simulink model "AD_Terry_VV"  (R2020b)
settings: Solver=VariableStepAuto  StartTime=0.0  StopTime=10.0  RelTol=1e-3
values from neighbouring files (symbols this model uses):
  A_2 = zeros(3)    [ANGULARTUNEVERSION2_VandV.m]
  B_2 = I_inv    [ANGULARTUNEVERSION2_VandV.m]
  C_2 = eye(3)    [ANGULARTUNEVERSION2_VandV.m]
  C_D = 0.6    [ANGULARTUNEVERSION2_VandV.m]    (also in Drag_Model_VV.m)
  constant_v = 1    [ANGULARTUNEVERSION2_VandV.m]
  D_2 = zeros(3)    [ANGULARTUNEVERSION2_VandV.m]
  rho = 1.225    [ANGULARTUNEVERSION2_VandV.m]    (also in Drag_Model_VV.m)
  S = 1*1.8    (= 1.8)    [ANGULARTUNEVERSION2_VandV.m]    (also in Drag_Model_VV.m = 2.5)
  sine_v = 0    [ANGULARTUNEVERSION2_VandV.m]
  T = 10.5    [ANGULARTUNEVERSION2_VandV.m]
  theta_wanted = [pi/2; 0; 0]    [ANGULARTUNEVERSION2_VandV.m]
  v_vehicle = [20; 10; 0]    [ANGULARTUNEVERSION2_VandV.m]    (also in Drag_Model_VV.m = [2;3;4])
  x_amp = 10    [ANGULARTUNEVERSION2_VandV.m]
  x_cp = [0.3; 0.2; 0.4]    [ANGULARTUNEVERSION2_VandV.m]
  x_freq = 1    [ANGULARTUNEVERSION2_VandV.m]
  y_amp = 15    [ANGULARTUNEVERSION2_VandV.m]
  y_freq = 1    [ANGULARTUNEVERSION2_VandV.m]
  z_amp = 5    [ANGULARTUNEVERSION2_VandV.m]
  z_freq = 1    [ANGULARTUNEVERSION2_VandV.m]
libraries: mpclib x1, fuzblock x1, cstblocks x1
settings Model: Creator=Jonathan van Zyl  LastModifiedBy=Jonathan van Zyl

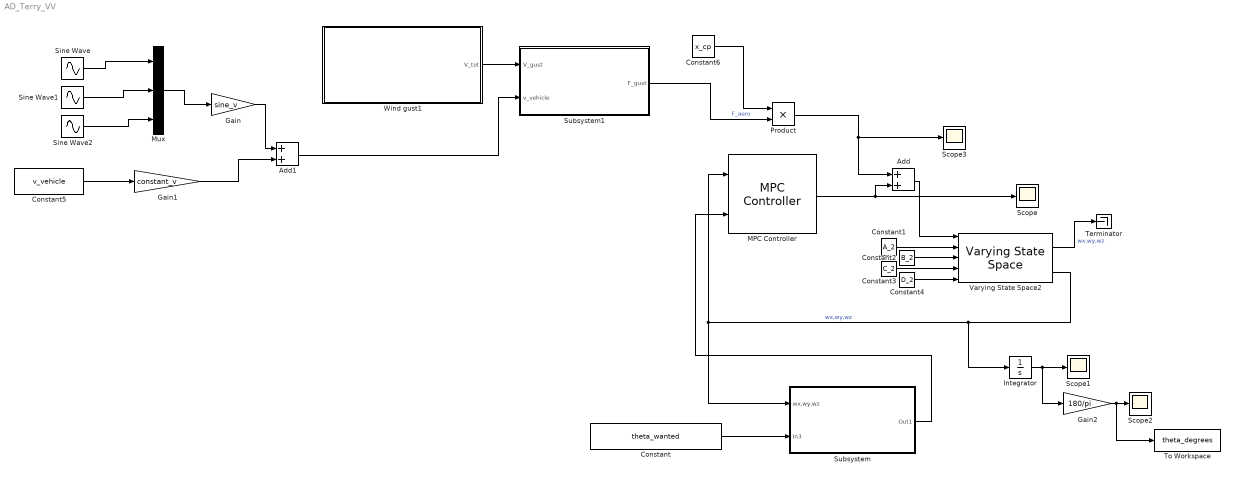
== system AD_Terry_VV ==
  Add : Sum
  Add1 : Sum
  Constant : Constant  Value=theta_wanted
  Constant1 : Constant  Value=A_2
  Constant2 : Constant  Value=B_2
  Constant3 : Constant  Value=C_2
  Constant4 : Constant  Value=D_2
  Constant5 : Constant  Value=v_vehicle
  Constant6 : Constant  Value=x_cp
  Gain : Gain  Gain=sine_v
  Gain1 : Gain  Gain=constant_v
  Gain2 : Gain  Gain=180/pi
  Integrator : Integrator
  MPC Controller : mpclib/MPC Controller  SCDEnableBlockLinearizationSpecification=on  mpcobj=MPCDesignerSession.AppData.Controllers.MPC  is_multiple=0  enable_value=0  return_u0=off  updateMPCinCallerWorkspace=on  md_inport=off  mv_inport=off  uref_inport=off  return_cost=off  return_mvseq=off  return_qpstatus=off  return_xseq=off  return_state=off  return_ovseq=off  state_inport=off  umin_inport=off  umax_inport=off  ymin_inport=off  ymax_inport=off  cc_inport=off  ywt_inport=off  uwt_inport=off  duwt_inport=off  rhoeps_inport=off  pm_inport=off  MaximumP=10  HorizonChoice=FixedHorizon  n_ts=0.1  n_p=10  n_mv=3  n_md=0  n_ud=0  n_mo=3  n_uo=0  BlockDataType=double  SampleTimeInherited=off  switch_inport=off
  Mux : Mux  Inputs=3
  Product : Product
  Scope{,1..3} (4 alike) : Scope
  Sine Wave : Sin  Amplitude=x_amp  Frequency=x_freq  SampleTime=0
  Sine Wave1 : Sin  Amplitude=y_amp  Frequency=y_freq  SampleTime=0
  Sine Wave2 : Sin  Amplitude=z_amp  Frequency=z_freq  SampleTime=0
  Subsystem : Subsystem
  Subsystem1 : Subsystem
  Terminator : Terminator
  To Workspace : ToWorkspace  VariableName=theta_degrees  SaveFormat=Timeseries  SampleTime=-1
  Varying State Space2 : cstblocks/Linear Parameter Varying/Varying State Space  x0=0  xNames=''  OutputX=on  OutputDX=off
  Wind gust1 : Subsystem
  wires:
  Constant5/1 -> Gain1/1
  Gain1/1 -> Add1/2
  Sine Wave/1 -> Mux/1
  Sine Wave1/1 -> Mux/2
  Sine Wave2/1 -> Mux/3
  Mux/1 -> Gain/1
  Gain/1 -> Add1/1
  Constant6/1 -> Product/1
  Subsystem1/1(F_gust) -> Product/2  "F_aero"
  Wind gust1/1(V_tot) -> Subsystem1/1(V_gust)
  Constant/1 -> Subsystem/2(In3)
  Varying State Space2/2 -> Integrator/1, MPC Controller/1, Subsystem/1(wx,wy,wz)  "wx,wy,wz"
  Constant1/1 -> Varying State Space2/2
  Subsystem/1(Out1) -> MPC Controller/2
  Integrator/1 -> Gain2/1, Scope1/1
  Constant3/1 -> Varying State Space2/4
  Constant2/1 -> Varying State Space2/3
  Product/1 -> Scope3/1, Add/1
  Gain2/1 -> To Workspace/1, Scope2/1
  Varying State Space2/1 -> Terminator/1  "wx,wy,wz"
  Add1/1 -> Subsystem1/2(v_vehicle)
  MPC Controller/1 -> Scope/1, Add/2
  Add/1 -> Varying State Space2/1
  Constant4/1 -> Varying State Space2/5

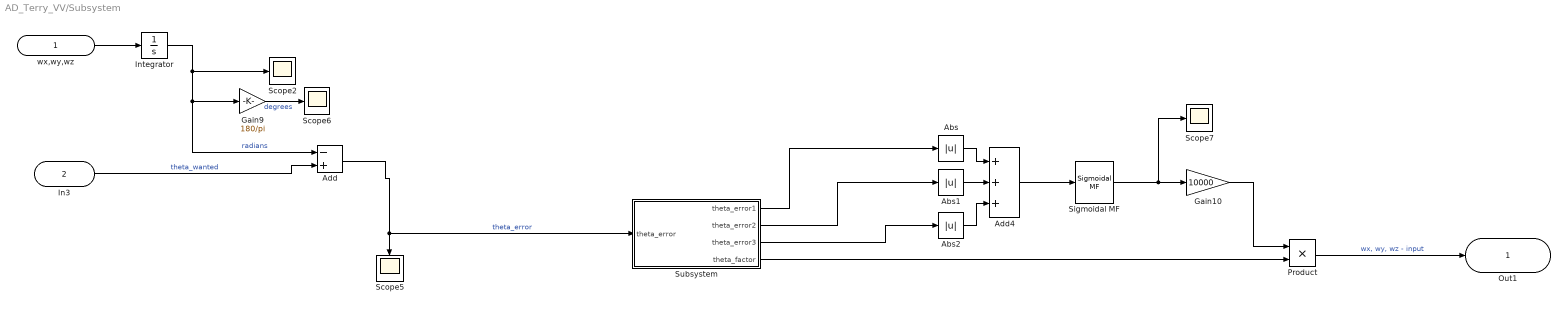
== system AD_Terry_VV/Subsystem ==
  wx,wy,wz : Inport
  In3 : Inport  Port=2
  Abs : Abs
  Abs1 : Abs
  Abs2 : Abs
  Add : Sum  Inputs=-+
  Add4 : Sum  Inputs=+++
  Gain10 : Gain  Gain=10000
  Gain9 : Gain  Gain=180/pi
  Integrator : Integrator
  Product : Product
  Scope{2,5..7} (4 alike) : Scope
  Sigmoidal MF : fuzblock/Membership  Functions/Sigmoidal MF  a=2.5  c=1.75
      settings: SourceProductBaseCode=FL
  Subsystem : Subsystem
  Out1 : Outport
  wires:
  Integrator/1 -> Add/1, Gain9/1, Scope2/1  "radians"
  Add/1 -> Subsystem/1(theta_error), Scope5/1  "theta_error"
  Abs2/1 -> Add4/3
  Abs1/1 -> Add4/2
  Gain9/1 -> Scope6/1  "degrees"
  Abs/1 -> Add4/1
  Gain10/1 -> Product/1
  Sigmoidal MF/1 -> Scope7/1, Gain10/1
  Add4/1 -> Sigmoidal MF/1
  In3/1 -> Add/2  "theta_wanted"
  Product/1 -> Out1/1  "wx, wy, wz - input"
  wx,wy,wz/1 -> Integrator/1
  Subsystem/1(theta_error1) -> Abs/1
  Subsystem/2(theta_error2) -> Abs1/1
  Subsystem/3(theta_error3) -> Abs2/1
  Subsystem/4(theta_factor) -> Product/2

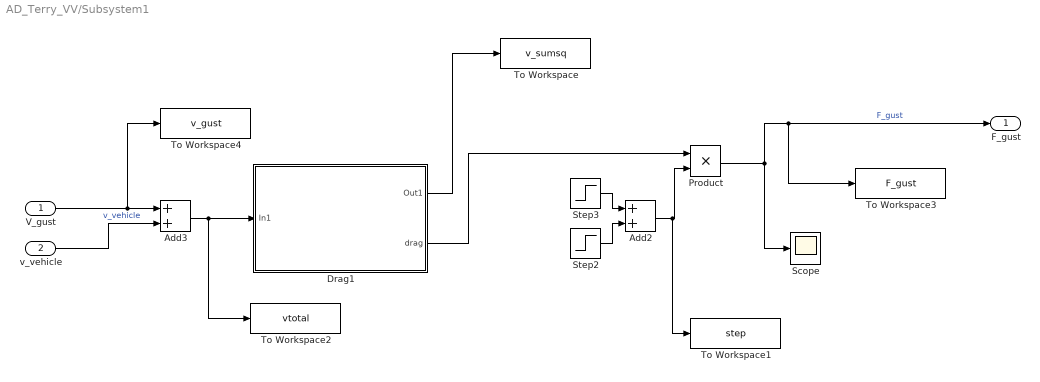
== system AD_Terry_VV/Subsystem1 ==
  V_gust : Inport
  v_vehicle : Inport  Port=2
  Add2 : Sum
  Add3 : Sum
  Drag1 : Subsystem
  Product : Product
  Scope : Scope
  Step2 : Step  Time=0  SampleTime=0
  Step3 : Step  Time=10.5  After=-1  SampleTime=0
  To Workspace : ToWorkspace  VariableName=v_sumsq  SampleTime=-1
  To Workspace1 : ToWorkspace  VariableName=step  SaveFormat=Timeseries  SampleTime=-1
  To Workspace2 : ToWorkspace  VariableName=vtotal  SaveFormat=Timeseries  SampleTime=-1
  To Workspace3 : ToWorkspace  VariableName=F_gust  SaveFormat=Timeseries  SampleTime=-1
  To Workspace4 : ToWorkspace  VariableName=v_gust  SaveFormat=Timeseries  SampleTime=-1
  F_gust : Outport
  wires:
  Product/1 -> F_gust/1, To Workspace3/1, Scope/1  "F_gust"
  Step3/1 -> Add2/1
  V_gust/1 -> To Workspace4/1, Add3/1
  Drag1/1(Out1) -> To Workspace/1
  Add3/1 -> Drag1/1(In1), To Workspace2/1
  Add2/1 -> To Workspace1/1, Product/2
  Step2/1 -> Add2/2
  v_vehicle/1 -> Add3/2  "v_vehicle"
  Drag1/2(drag) -> Product/1

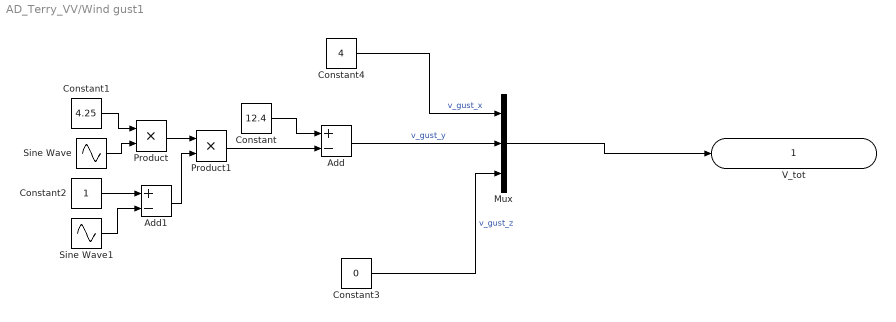
== system AD_Terry_VV/Wind gust1 ==
  Add : Sum  Inputs=+-
  Add1 : Sum  Inputs=+-
  Constant : Constant  Value=12.4
  Constant1 : Constant  Value=4.25
  Constant2 : Constant
  Constant3 : Constant  Value=0
  Constant4 : Constant  Value=4  VectorParams1D=off
  Mux : Mux  Inputs=3
  Product : Product
  Product1 : Product
  Sine Wave : Sin  Frequency=3*pi/T  SampleTime=0
  Sine Wave1 : Sin  Frequency=2*pi/T  Phase=pi/2  SampleTime=0
  V_tot : Outport
  wires:
  Constant/1 -> Add/1
  Constant1/1 -> Product/1
  Sine Wave/1 -> Product/2
  Constant2/1 -> Add1/1
  Sine Wave1/1 -> Add1/2
  Product/1 -> Product1/1
  Add1/1 -> Product1/2
  Product1/1 -> Add/2
  Add/1 -> Mux/2  "v_gust_y"
  Constant3/1 -> Mux/3  "v_gust_z"
  Mux/1 -> V_tot/1
  Constant4/1 -> Mux/1  "v_gust_x"

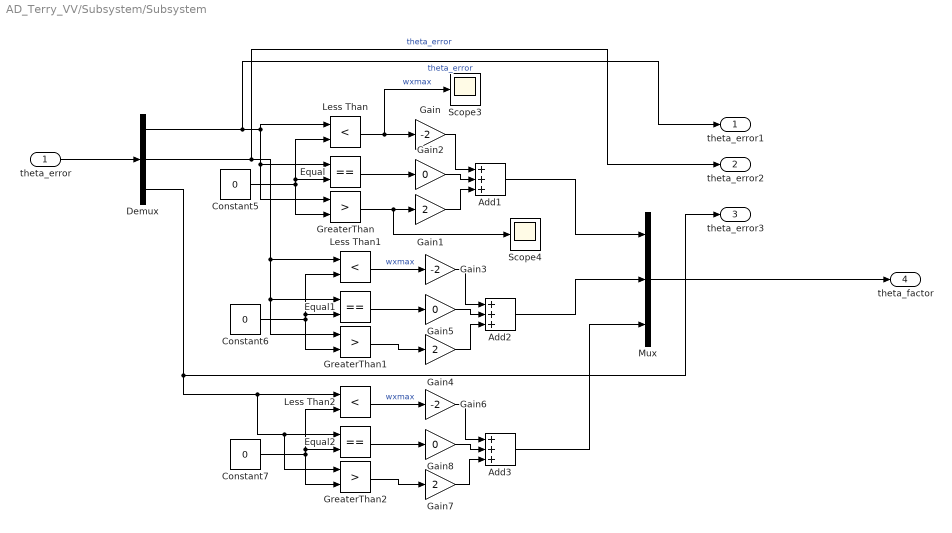
== system AD_Terry_VV/Subsystem/Subsystem ==
  theta_error : Inport
  Add1 : Sum  Inputs=+++
  Add2 : Sum  Inputs=+++
  Add3 : Sum  Inputs=+++
  Constant5 : Constant  Value=0
  Constant6 : Constant  Value=0
  Constant7 : Constant  Value=0
  Demux : Demux  Outputs=3
  Equal : RelationalOperator  Operator===  OutDataTypeStr=boolean  RndMeth=Simplest
  Equal1 : RelationalOperator  Operator===  OutDataTypeStr=boolean  RndMeth=Simplest
  Equal2 : RelationalOperator  Operator===  OutDataTypeStr=boolean  RndMeth=Simplest
  Gain : Gain  Gain=-2
  Gain1 : Gain  Gain=2
  Gain2 : Gain  Gain=0
  Gain3 : Gain  Gain=-2
  Gain4 : Gain  Gain=2
  Gain5 : Gain  Gain=0
  Gain6 : Gain  Gain=-2
  Gain7 : Gain  Gain=2
  Gain8 : Gain  Gain=0
  GreaterThan : RelationalOperator  Operator=>  OutDataTypeStr=boolean  RndMeth=Simplest
  GreaterThan1 : RelationalOperator  Operator=>  OutDataTypeStr=boolean  RndMeth=Simplest
  GreaterThan2 : RelationalOperator  Operator=>  OutDataTypeStr=boolean  RndMeth=Simplest
  Less Than : RelationalOperator  Operator=<  OutDataTypeStr=boolean  RndMeth=Simplest
  Less Than1 : RelationalOperator  Operator=<  OutDataTypeStr=boolean  RndMeth=Simplest
  Less Than2 : RelationalOperator  Operator=<  OutDataTypeStr=boolean  RndMeth=Simplest
  Mux : Mux  Inputs=3
  Scope3 : Scope
  Scope4 : Scope
  theta_error1 : Outport
  theta_error2 : Outport  Port=2
  theta_error3 : Outport  Port=3
  theta_factor : Outport  Port=4
  wires:
  Add1/1 -> Mux/1
  Constant5/1 -> Equal/2, Less Than/2, GreaterThan/2
  Equal2/1 -> Gain8/1
  Demux/1 -> theta_error1/1, GreaterThan/1, Equal/1, Less Than/1  "theta_error"
  GreaterThan2/1 -> Gain7/1
  Gain1/1 -> Add1/3
  Gain7/1 -> Add3/3
  Less Than1/1 -> Gain3/1  "wxmax"
  Gain6/1 -> Add3/1
  Equal/1 -> Gain2/1
  Gain5/1 -> Add2/2
  Add3/1 -> Mux/3
  GreaterThan/1 -> Scope4/1, Gain1/1
  Constant6/1 -> Equal1/2, Less Than1/2, GreaterThan1/2
  Demux/3 -> theta_error3/1, GreaterThan2/1, Equal2/1, Less Than2/1
  Gain3/1 -> Add2/1
  Constant7/1 -> Equal2/2, Less Than2/2, GreaterThan2/2
  Equal1/1 -> Gain5/1
  Gain8/1 -> Add3/2
  Gain4/1 -> Add2/3
  GreaterThan1/1 -> Gain4/1
  Gain/1 -> Add1/1
  Demux/2 -> theta_error2/1, GreaterThan1/1, Equal1/1, Less Than1/1  "theta_error"
  Gain2/1 -> Add1/2
  Add2/1 -> Mux/2
  Less Than/1 -> Scope3/1, Gain/1  "wxmax"
  Less Than2/1 -> Gain6/1  "wxmax"
  theta_error/1 -> Demux/1
  Mux/1 -> theta_factor/1

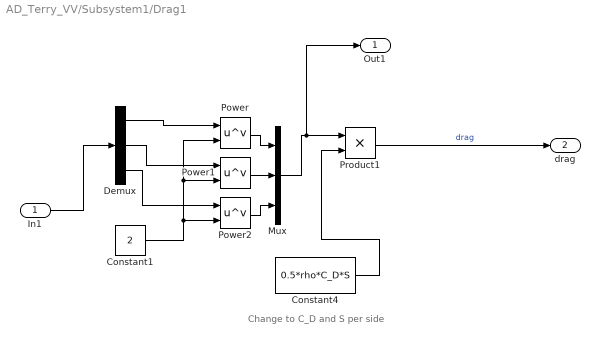
== system AD_Terry_VV/Subsystem1/Drag1 ==
  note: Change to C_D and S per side
  In1 : Inport
  Constant1 : Constant  Value=2
  Constant4 : Constant  Value=0.5*rho*C_D*S
  Demux : Demux  Outputs=3
  Mux : Mux  Inputs=3
  Power : Math  Operator=pow  SaturateOnIntegerOverflow=on
  Power1 : Math  Operator=pow  SaturateOnIntegerOverflow=on
  Power2 : Math  Operator=pow  SaturateOnIntegerOverflow=on
  Product1 : Product
  Out1 : Outport
  drag : Outport  Port=2
  wires:
  Constant1/1 -> Power2/2, Power1/2, Power/2
  Power2/1 -> Mux/3
  Power/1 -> Mux/1
  In1/1 -> Demux/1
  Demux/1 -> Power/1
  Demux/3 -> Power2/1
  Demux/2 -> Power1/1
  Power1/1 -> Mux/2
  Constant4/1 -> Product1/2
  Mux/1 -> Out1/1, Product1/1
  Product1/1 -> drag/1  "drag"
